simulink model "system_response"  (Simulink 7.9)
settings: Solver=ode3  StartTime=0.0  StopTime=15  FixedStep=0.05  RelTol=1e-3
values from neighbouring files (symbols this model uses):
  sx_d = [time sx_d]    [WPG_results.m]    (also in WPG_sim.m; control_layer_zmp_com_init.m = [time sx_d_y]; control_layer_zmp_com_init_2.m = [time sx_d_x])
settings Model: Creator=pajon  LastModifiedBy=pajon

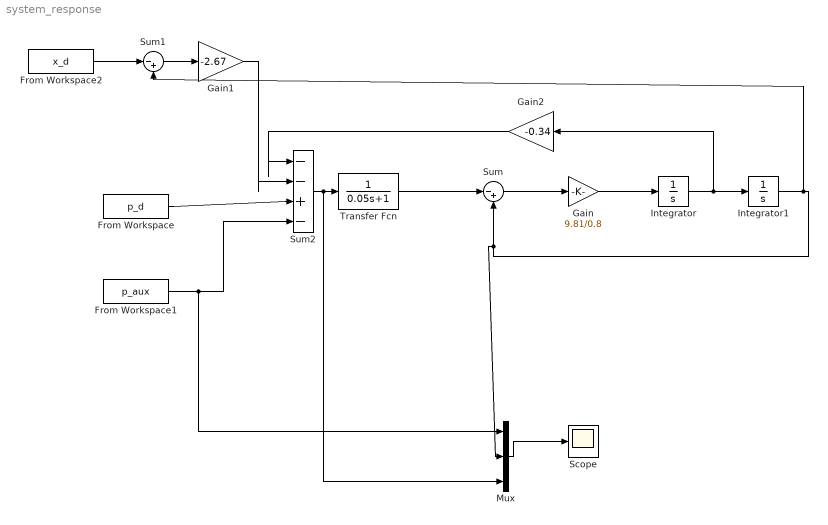
== system system_response ==
  From Workspace : FromWorkspace  VariableName=p_d  SampleTime=0
  From Workspace1 : FromWorkspace  VariableName=p_aux  SampleTime=0
  From Workspace2 : FromWorkspace  VariableName=x_d  SampleTime=0
  Gain : Gain  Gain=9.81/0.8
  Gain1 : Gain  Gain=-2.67
  Gain2 : Gain  Gain=-0.34
  Integrator : Integrator  InitialCondition=sx_d(1,2)
  Integrator1 : Integrator  InitialCondition=sx_d(1,2)
  Mux : Mux  Inputs=3
  Scope : Scope
  Sum : Sum  Inputs=|-+
  Sum1 : Sum  Inputs=|-+
  Sum2 : Sum  Inputs=|--+-
  Transfer Fcn : TransferFcn  Denominator=[0.05 1]
  wires:
  Transfer Fcn/1 -> Sum/1
  Sum/1 -> Gain/1
  Gain/1 -> Integrator/1
  Integrator/1 -> Integrator1/1, Gain2/1
  Integrator1/1 -> Sum1/2, Sum/2, Mux/2
  From Workspace2/1 -> Sum1/1
  Sum1/1 -> Gain1/1
  From Workspace/1 -> Sum2/3
  From Workspace1/1 -> Sum2/4, Mux/1
  Gain1/1 -> Sum2/2
  Gain2/1 -> Sum2/1
  Sum2/1 -> Transfer Fcn/1, Mux/3
  Mux/1 -> Scope/1
